simulink model "test2_Pace_UART"  (R2017b)
settings: Solver=FixedStepAuto  StartTime=0.0  StopTime=inf  FixedStep=1e-3  RelTol=1e-3  EnableMultiTasking=on
undefined symbols (not defined in the file): D0, D1, D10, D11, D12, D13, D2, D3, D5, D6, D8, D9, PTA0, PTA1, PTA2, PTB9, PTC16, PTC17, PTC2, PTC4, PTD0, PTD1, PTD2, PTD3
libraries: frdmk64flib x17, etargetslib x3
settings Model: ExtModeTrigDuration=5  Creator=zhuh30  LastModifiedBy=Michael
settings OptimizationCC: PassReuseOutputArgsAs=Individual arguments  MaxStackSize=64
settings DebuggingCC: ParameterTunabilityLossMsg=error
settings HardwareCC: ProdBitPerPointer=32  ProdBitPerSizeT=32  ProdBitPerPtrDiffT=32  ProdLargestAtomicInteger=Long  ProdLargestAtomicFloat=Double  ProdWordSize=32  ProdHWDeviceType=ARM Compatible->ARM Cortex
settings SFSimCC: MATLABDynamicMemAlloc=off
settings RTWCC: SystemTargetFile=ert.tlc  HardwareBoard=NXP FRDM-K64F  TemplateMakefile=ert_default_tmf  GenerateReport=on  Toolchain=GNU Tools for ARM Embedded Processors  IncludeHyperlinkInReport=on  LaunchReport=on  GenerateTraceInfo=on  GenerateTraceReport=on  GenerateTraceReportSl=on  GenerateTraceReportSf=on  GenerateTraceReportEml=on
settings CodeAppCC: ForceParamTrailComments=on  IgnoreCustomStorageClasses=off  OperatorAnnotations=on  SimulinkDataObjDesc=on  SFDataObjDesc=on  InsertBlockDesc=on

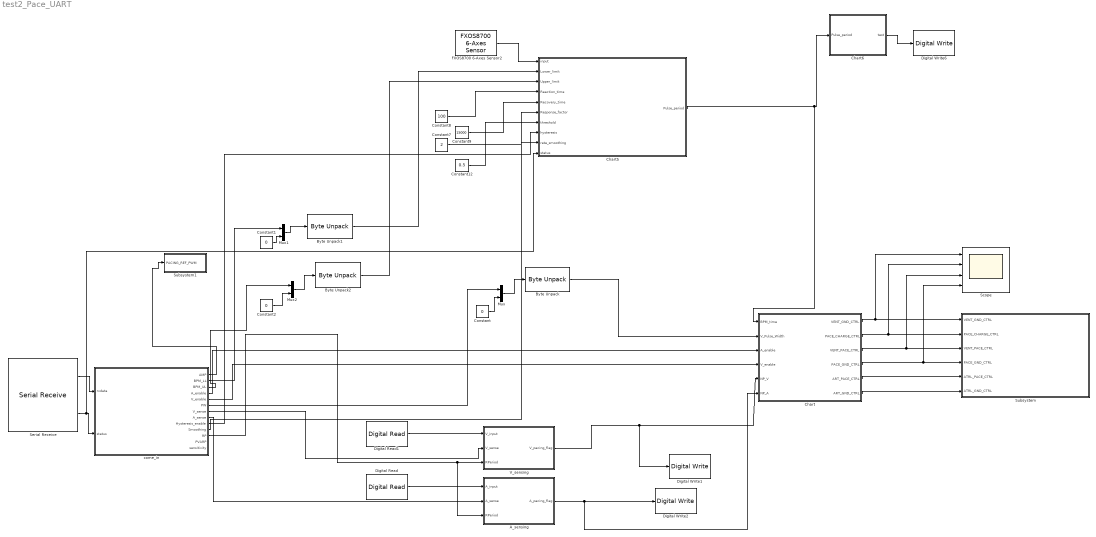
== system test2_Pace_UART ==
  A_sensing : Stateflow chart  TreatAsAtomicUnit=on
  Byte Unpack : etargetslib/Byte Unpack  dimensions={[1]}  datatypes={'uint16'}  byteAlign=1
  Byte Unpack1 : etargetslib/Byte Unpack  dimensions={[1]}  datatypes={'uint16'}  byteAlign=1
  Byte Unpack2 : etargetslib/Byte Unpack  dimensions={[1]}  datatypes={'uint16'}  byteAlign=1
  Chart : Stateflow chart  TreatAsAtomicUnit=on
  Chart5 : Stateflow chart  TreatAsAtomicUnit=on
  Chart6 : Stateflow chart  TreatAsAtomicUnit=on
  Constant : Constant  Value=0  OutDataTypeStr=uint8
  Constant1 : Constant  Value=0  OutDataTypeStr=uint8
  Constant12 : Constant  Value=0.5
  Constant2 : Constant  Value=0  OutDataTypeStr=uint8
  Constant7 : Constant  Value=2
  Constant8 : Constant  Value=100
  Constant9 : Constant  Value=15000
  Digital Read : frdmk64flib/Digital Read  Whichpin=PTC16 (D0)  SampleTime=-1
      settings: SourceProductName=Simulink Coder Support Package for NXP FRDM-K64F Board
  Digital Read1 : frdmk64flib/Digital Read  Whichpin=PTC17 (D1)  SampleTime=-1
      settings: SourceProductName=Simulink Coder Support Package for NXP FRDM-K64F Board
  Digital Write1 : frdmk64flib/Digital Write  Whichpin=RED_LED
      settings: SourceProductName=Simulink Coder Support Package for NXP FRDM-K64F Board
  Digital Write2 : frdmk64flib/Digital Write  Whichpin=BLUE_LED
      settings: SourceProductName=Simulink Coder Support Package for NXP FRDM-K64F Board
  Digital Write6 : frdmk64flib/Digital Write  Whichpin=GREEN_LED
      settings: SourceProductName=Simulink Coder Support Package for NXP FRDM-K64F Board
  FXOS8700 6-Axes Sensor2 : frdmk64flib/FXOS8700 6-Axes Sensor  Activesensor=Accelerometer only  ODR=800Hz  HybridODR=400Hz  Accelfullrange=-4g to +4g  SampleTime=-1
      settings: SourceProductName=Simulink Coder Support Package for NXP FRDM-K64F Board
  Mux : Mux  Inputs=2
  Mux1 : Mux  Inputs=2
  Mux2 : Mux  Inputs=2
  Scope : Scope  NumInputPorts=4
  Serial Receive : frdmk64flib/Serial Receive  SCIModule=0  Baudrate=uint32(9600)  Parity=None  StopBits=1  HardwareFlowControl=None  ByteOrder=LittleEndian  DataType=uint8  DataLength=15  BlockingMode=off  OutputStatus=on  SampleTime=-1
      settings: SourceProductName=Simulink Coder Support Package for NXP FRDM-K64F Board
  Subsystem : Subsystem
  Subsystem1 : Subsystem
  V_sensing : Stateflow chart  TreatAsAtomicUnit=on
  come_in : Stateflow chart  TreatAsAtomicUnit=on
  wires:
  come_in/1(AMP) -> Subsystem1/1(PACING_REF_PWM)
  Serial Receive/1 -> come_in/1(rxdata)
  Serial Receive/2 -> Chart5/10(status), come_in/2(status)
  come_in/2(BPM_LL) -> Mux1/1
  come_in/3(BPM_UL) -> Mux2/1
  come_in/6(PW) -> Mux/1
  Constant/1 -> Mux/2
  Mux/1 -> Byte Unpack/1
  Mux1/1 -> Byte Unpack1/1
  Constant1/1 -> Mux1/2
  Mux2/1 -> Byte Unpack2/1
  Constant2/1 -> Mux2/2
  V_sensing/1(V_pacing_flag) -> Digital Write1/1, Chart/5(NP_V)
  Digital Read/1 -> A_sensing/1(A_input)
  A_sensing/1(A_pacing_flag) -> Chart/6(NP_A), Digital Write2/1
  come_in/7(V_sense) -> V_sensing/2(V_sense)
  come_in/8(A_sense) -> A_sensing/2(A_sense)
  come_in/11(RP) -> A_sensing/3(RPeriod), V_sensing/3(RPeriod)
  Chart/5(ART_PACE_CTRL) -> Subsystem/5(ATRL_PACE_CTRL)
  Chart/3(VENT_PACE_CTRL) -> Scope/3, Subsystem/3(VENT_PACE_CTRL)
  Chart/6(ART_GND_CTRL) -> Subsystem/6(ATRL_GND_CTRL)
  Chart/1(VENT_GND_CTRL) -> Scope/1, Subsystem/1(VENT_GND_CTRL)
  Chart/2(PACE_CHARGE_CTRL) -> Scope/2, Subsystem/2(PACE_CHARGE_CTRL)
  Byte Unpack/1 -> Chart/2(V_Pulse_Width)
  Chart/4(PACE_GND_CTRL) -> Scope/4, Subsystem/4(PACE_GND_CTRL)
  Digital Read1/1 -> V_sensing/1(V_input)
  Byte Unpack2/1 -> Chart5/3(Upper_limit)
  FXOS8700 6-Axes Sensor2/1 -> Chart5/1(input)
  Constant12/1 -> Chart5/7(threshold)
  Byte Unpack1/1 -> Chart5/2(Lower_limit)
  Chart6/1(test) -> Digital Write6/1
  Constant9/1 -> Chart5/5(Recovery_time)
  Constant8/1 -> Chart5/4(Reaction_time)
  Constant7/1 -> Chart5/6(Response_factor)
  come_in/5(V_enable) -> Chart/4(V_enable)
  come_in/4(A_enable) -> Chart/3(A_enable)
  Chart5/1(Pulse_period) -> Chart/1(BPM_time), Chart6/1(Pulse_period)
  come_in/9(Hysteresis_enable) -> Chart5/8(hysteresis)
  come_in/10(Smoothing) -> Chart5/9(rate_smoothing)

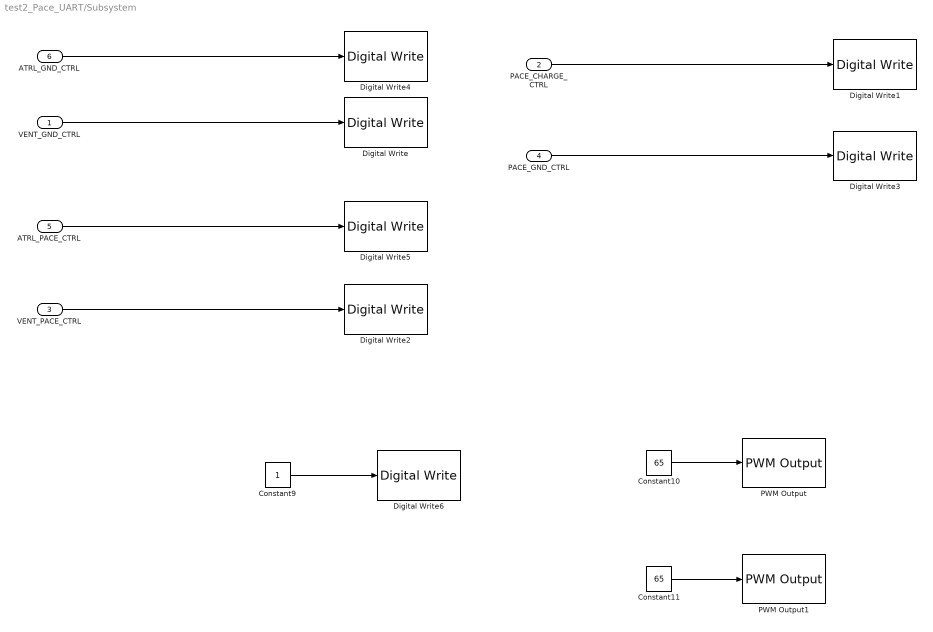
== system test2_Pace_UART/Subsystem ==
  VENT_GND_CTRL : Inport
  PACE_CHARGE_CTRL : Inport  Port=2
  VENT_PACE_CTRL : Inport  Port=3
  PACE_GND_CTRL : Inport  Port=4
  ATRL_PACE_CTRL : Inport  Port=5
  ATRL_GND_CTRL : Inport  Port=6
  Constant10 : Constant  Value=65
  Constant11 : Constant  Value=65
  Constant9 : Constant
  Digital Write : frdmk64flib/Digital Write  Whichpin=PTD3 (D12)
      settings: SourceProductName=Simulink Coder Support Package for NXP FRDM-K64F Board
  Digital Write1 : frdmk64flib/Digital Write  Whichpin=PTB9 (D2)
      settings: SourceProductName=Simulink Coder Support Package for NXP FRDM-K64F Board
  Digital Write2 : frdmk64flib/Digital Write  Whichpin=PTC4 (D9)
      settings: SourceProductName=Simulink Coder Support Package for NXP FRDM-K64F Board
  Digital Write3 : frdmk64flib/Digital Write  Whichpin=PTD0 (D10)
      settings: SourceProductName=Simulink Coder Support Package for NXP FRDM-K64F Board
  Digital Write4 : frdmk64flib/Digital Write  Whichpin=PTD2 (D11)
      settings: SourceProductName=Simulink Coder Support Package for NXP FRDM-K64F Board
  Digital Write5 : frdmk64flib/Digital Write  Whichpin=PTA0 (D8)
      settings: SourceProductName=Simulink Coder Support Package for NXP FRDM-K64F Board
  Digital Write6 : frdmk64flib/Digital Write  Whichpin=PTD1 (D13)
      settings: SourceProductName=Simulink Coder Support Package for NXP FRDM-K64F Board
  PWM Output : frdmk64flib/PWM Output  Whichpin=PTC2 (D6)  InitialFrequency=916  InitialDutyCycle=60
      settings: SourceProductName=Simulink Coder Support Package for NXP FRDM-K64F Board
  PWM Output1 : frdmk64flib/PWM Output  Whichpin=PTA1 (D3)  InitialFrequency=916  InitialDutyCycle=60
      settings: SourceProductName=Simulink Coder Support Package for NXP FRDM-K64F Board
  wires:
  VENT_GND_CTRL/1 -> Digital Write/1
  PACE_CHARGE_CTRL/1 -> Digital Write1/1
  VENT_PACE_CTRL/1 -> Digital Write2/1
  PACE_GND_CTRL/1 -> Digital Write3/1
  ATRL_GND_CTRL/1 -> Digital Write4/1
  ATRL_PACE_CTRL/1 -> Digital Write5/1
  Constant9/1 -> Digital Write6/1
  Constant10/1 -> PWM Output/1
  Constant11/1 -> PWM Output1/1

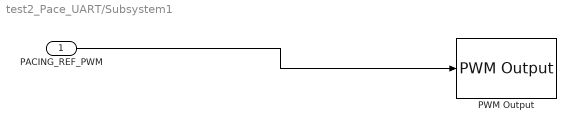
== system test2_Pace_UART/Subsystem1 ==
  PACING_REF_PWM : Inport
  PWM Output : frdmk64flib/PWM Output  Whichpin=PTA2 (D5)  InitialFrequency=916  InitialDutyCycle=0
      settings: SourceProductName=Simulink Coder Support Package for NXP FRDM-K64F Board
  wires:
  PACING_REF_PWM/1 -> PWM Output/1

== stateflow chart test2_Pace_UART/come_in ==
  state SET_RARAM [commented out]
    entry:
    BPM_UL = rxdata(3);
    BPM_LL = rxdata(4);
    AMP = rxdata(5);
    PW = rxdata(6);
  state INITIAL [commented out]
    entry:
    BPM_UL = 60;
    BPM_LL = 60;
    AMP = 60;
    PW = 100;
    A_enable = 1;
    V_enable = 0;
    A_sense = 1;
    V_sense = 0;
    RP = 500;
    Hysteresis_enable = 0;
    Smoothing = 0;
    PVARP = 0;
  state STANDBY [commented out]
  state SET_RARAM1
    entry:
    BPM_LL = rxdata(3);
    BPM_UL = rxdata(4);
    AMP = rxdata(5);
    PW = rxdata(6);
    if (rxdata(7) == hex2dec('1'))
    A_enable = 1;
    V_enable = 0;
    V_sense= 0;
    A_sense = rxdata(8);
    sensitivity = rxdata(9);
    RP = 10* typecast(rxdata(10:11), 'uint16');
    Hysteresis_enable = rxdata(12);
    Smoothing = rxdata(13);
    PVARP = typecast(rxdata(14:15), 'uint16');
    elseif (rxdata(7) == hex2dec('0'))
    A_enable = 0;
    V_enable = 1;
    A_sense= 0;
    V_sense = rxdata(8);
    sensitivity = rxdata(9);
    RP = 10*typecast(rxdata(10:11), 'uint16');
    Hysteresis_enable = rxdata(12);
    Smoothing = rxdata(13);
    PVARP = typecast(rxdata(14:15), 'uint16');
    else
    A_enable = 0;
    V_enable = 0;
    A_sense= 0;
    V_sense = rxdata(8);
    sensitivity = rxdata(9);
    RP = 10*typecast(rxdata(10:11), 'uint16');
    Hysteresis_enable = rxdata(12);
    Smoothing = rxdata(13);
    PVARP = typecast(rxdata(14:15), 'uint16');
    end
  state VOO_or_VVI [commented out]
    entry:
    A_enable = 0;
    V_enable = 1;
    A_sense = 0;
    V_sense = rxdata(8);
    sensitivity = rxdata(9);
    RP = 10*typecast(rxdata(10:11), 'uint16');
    Hysteresis_enable = rxdata(12);
    Smoothing = rxdata(13);
    PVARP = typecast(rxdata(14:15), 'uint16');
  state AOO_or_AAI [commented out]
    entry:
    A_enable = 1;
    V_enable = 0;
    V_sense = 0;
    A_sense = rxdata(8);
    sensitivity = rxdata(9);
    RP = 10* typecast(rxdata(10:11), 'uint16');
    Hysteresis_enable = rxdata(12);
    Smoothing = rxdata(13);
    PVARP = typecast(rxdata(14:15), 'uint16');
  state INITIAL1
    entry:
    BPM_UL = 120;
    BPM_LL = 60;
    AMP = 60;
    PW = 100;
    A_enable = 1;
    V_enable = 0;
    A_sense = 1;
    V_sense = 0;
    RP = 50;
    Hysteresis_enable = 0;
    Smoothing = 0;
    PVARP = 0;
  state STANDBY1
  SET_RARAM -> STANDBY [commented out]
  (junction 6) -> STANDBY [commented out]
  (default) -> INITIAL [commented out]
  INITIAL -> STANDBY [commented out]
  STANDBY -> (junction 6) [commented out] : [status == 0]
  (junction 6) -> (junction 7) [commented out] : [rxdata(1) == hex2dec('16')]
  (junction 7) -> SET_RARAM [commented out] : [rxdata(2) == hex2dec('55')]
  (junction 7) -> STANDBY [commented out]
  VOO_or_VVI -> STANDBY [commented out]
  AOO_or_AAI -> STANDBY [commented out]
  SET_RARAM -> AOO_or_AAI [commented out] : [rxdata(7) == hex2dec('1')]
  SET_RARAM -> VOO_or_VVI [commented out] : [rxdata(7) == hex2dec('0')]
  (junction 55) -> STANDBY1 [order 2]
  (default) -> INITIAL1
  INITIAL1 -> STANDBY1
  STANDBY1 -> (junction 55) : [status == 0]
  (junction 55) -> (junction 63) [order 1] : [rxdata(1) == hex2dec('16')]
  (junction 63) -> SET_RARAM1 [order 1] : [rxdata(2) == hex2dec('55')]
  (junction 63) -> STANDBY1 [order 2]
  SET_RARAM1 -> STANDBY1
  data: AMP output uint8; rxdata input uint8; status input uint8; BPM_LL output uint8; BPM_UL output uint8; A_enable output uint8; V_enable output uint8; PW output uint8; V_sense output uint8; A_sense output uint8; Hysteresis_enable output uint8; Smoothing output uint8; RP output uint16; PVARP output uint16; sensitivity output uint8

== stateflow chart test2_Pace_UART/A_sensing ==
  state SENSING_A_wait
    entry:
    A_pacing_flag = 0;
  state A_pace_sensed
    entry:
    A_pacing_flag = 1;
  SENSING_A_wait -> A_pace_sensed [order 2] : [A_input == 1]
  (default) -> SENSING_A_wait
  A_pace_sensed -> SENSING_A_wait : after(RPeriod,msec)
  SENSING_A_wait -> SENSING_A_wait [order 1] : [A_sense == 0]
  data: A_input input; A_pacing_flag output uint8; A_sense input; RPeriod input

== stateflow chart test2_Pace_UART/Chart ==
  state Initial_state
    entry:
    ART_PACE_CTRL = false;
    ART_GND_CTRL = true
    VENT_PACE_CTRL = false;
    VENT_GND_CTRL = true;
    PACE_CHARGE_CTRL = true;
    PACE_GND_CTRL = true;
  state Charging_state_V
    entry:
    PACE_CHARGE_CTRL = true;
    VENT_PACE_CTRL = false;
    VENT_GND_CTRL = true;
    PACE_GND_CTRL = true;
    ART_PACE_CTRL = false;
    ART_GND_CTRL = true;
  state Charging_state_A
    entry:
    PACE_CHARGE_CTRL = true;
    ART_PACE_CTRL = false;
    ART_GND_CTRL = true;
    PACE_GND_CTRL = true;
    VENT_PACE_CTRL = false;
    VENT_GND_CTRL = true;
  state Delay_state_A
    entry:
    PACE_CHARGE_CTRL = true;
    ART_PACE_CTRL = false;
    ART_GND_CTRL = true;
    PACE_GND_CTRL = true;
    VENT_PACE_CTRL = false;
    VENT_GND_CTRL = true;
  state Delay_state_V
    entry:
    PACE_CHARGE_CTRL = true;
    VENT_PACE_CTRL = false;
    VENT_GND_CTRL = true;
    PACE_GND_CTRL = true;
    ART_PACE_CTRL = false;
    ART_GND_CTRL = true;
  state Pacing_state_V
    entry:
    PACE_CHARGE_CTRL = false;
    VENT_PACE_CTRL = true;
    VENT_GND_CTRL = false;
    PACE_GND_CTRL = true;
    ART_PACE_CTRL = false;
    ART_GND_CTRL = true;
  state Pacing_state
    entry:
    PACE_CHARGE_CTRL = false;
    ART_PACE_CTRL = true;
    ART_GND_CTRL = false;
    PACE_GND_CTRL = true;
    VENT_PACE_CTRL = false;
    VENT_GND_CTRL = true;
  (default) -> Initial_state
  Initial_state -> Charging_state_V [order 1] : [V_enable == 1]
  Initial_state -> Charging_state_A [order 2] : [A_enable == 1]
  Charging_state_A -> Delay_state_A [order 2] : [NP_A == 1]
  Charging_state_V -> Delay_state_V [order 2] : [NP_V == 1]
  Charging_state_V -> Charging_state_A [order 3] : [A_enable == 1]
  Delay_state_A -> Delay_state_A [order 1] : [NP_A == 1]
  Charging_state_A -> Charging_state_V [order 3] : [V_enable == 1]
  Delay_state_V -> Delay_state_V [order 1] : [NP_V == 1]
  Pacing_state -> Charging_state_A [order 1] : after(V_Pulse_Width,msec)
  Pacing_state_V -> Charging_state_V [order 1] : after(V_Pulse_Width,msec)
  Charging_state_V -> Pacing_state_V [order 1] : after(BPM_time-V_Pulse_Width,msec)
  Charging_state_A -> Pacing_state [order 1] : after(BPM_time-V_Pulse_Width,msec)
  Delay_state_A -> Pacing_state [order 2] : after(BPM_time,msec)
  Pacing_state -> Delay_state_A [order 2] : [NP_A == 1]
  Delay_state_V -> Pacing_state_V [order 2] : after(BPM_time,msec)
  Pacing_state_V -> Delay_state_V [order 2] : [NP_V == 1]
  data: BPM_time input; VENT_GND_CTRL output; PACE_CHARGE_CTRL output; VENT_PACE_CTRL output; PACE_GND_CTRL output; V_Pulse_Width input; A_enable input; V_enable input; ART_PACE_CTRL output; ART_GND_CTRL output; NP_V input; NP_A input

== stateflow chart test2_Pace_UART/V_sensing ==
  state SENSING_V_wait
    entry:
    V_pacing_flag = 0;
  state V_pacing_sensed
    entry:
    V_pacing_flag = 1;
  SENSING_V_wait -> V_pacing_sensed [order 2] : [V_input == 1]
  (default) -> SENSING_V_wait
  V_pacing_sensed -> SENSING_V_wait : after(RPeriod,msec)
  SENSING_V_wait -> SENSING_V_wait [order 1] : [V_sense == 0]
  data: V_input input; V_pacing_flag output uint8; V_sense input; RPeriod input

== stateflow chart test2_Pace_UART/Chart5 ==
  state Initial1
    entry:
    norm_xy = ((input(1)^2.0) + (input(2)^2.0))^(1/2);
    BPM = Lower_limit;
    Pulse_period = uint16(60000/BPM);
    counter_reaction = 0;
    counter_recovery = 0;
  state norm_over_state
    entry:
    norm_xy = ((input(1)^2.0) + (input(2)^2.0))^(1/2);
    counter_reaction = counter_reaction + 1;
    counter_recovery = 0;
    counter_update_increase = 0;
  state norm_below_state
    entry:
    if (BPM > (Lower_limit + Upper_limit)/2)
    BPM = BPM - Response_factor;
    else
    BPM = Lower_limit;
    end
    Pulse_period = uint16(60000/BPM);
    norm_xy = ((input(1)^2.0) + (input(2)^2.0))^(1/2);
    counter_update = 0;
    counter_reaction = 0;
    counter_recovery = counter_recovery + 1;
  state update_input
    entry:
    norm_xy = ((input(1)^2.0) + (input(2)^2.0))^(1/2);
    counter_update = counter_update + 1;
    counter_update_increase = 0;
  state update_input_increase
    entry:
    norm_xy = ((input(1)^2.0) + (input(2)^2.0))^(1/2);
    counter_update_increase=counter_update_increase + 1;
  state Increase_rate
    entry:
    if (BPM < Upper_limit)
    BPM = BPM + Response_factor;
    else
    BPM = Upper_limit;
    end
    Pulse_period = uint16(60000/BPM);
    norm_xy = ((input(1)^2.0) + (input(2)^2.0))^(1/2);
    counter_reaction = 0;
    counter_update_increase = 0;
    counter_update = 0;
    counter_recovery = 0;
  Initial1 -> Initial1 [order 2] : after(1,msec)
  (default) -> Initial1
  Initial1 -> norm_over_state [order 1] : [norm_xy>threshold]
  norm_below_state -> Initial1 [order 2] : [counter_recovery >= 30]
  norm_over_state -> Initial1 [order 2] : [norm_xy <= threshold]
  norm_below_state -> Initial1 [order 1] : [status == 0]
  norm_over_state -> Initial1 [order 1] : [status == 0]
  update_input_increase -> Initial1 [order 1] : [status == 0]
  Increase_rate -> Initial1 [order 1] : [status == 0]
  update_input -> Initial1 [order 1] : [status == 0]
  norm_over_state -> norm_over_state [order 4] : after(1,msec)
  norm_below_state -> norm_over_state [order 3] : [norm_xy > threshold]
  update_input -> norm_over_state [order 4] : [norm_xy > threshold]
  norm_over_state -> update_input_increase [order 3] : [counter_reaction >= Reaction_time]
  norm_below_state -> update_input [order 4] : [norm_xy <= threshold]
  update_input -> norm_below_state [order 2] : [counter_update >= Recovery_time/30]
  update_input_increase -> update_input [order 3] : [norm_xy <= threshold]
  update_input -> update_input [order 3] : after(1,msec)
  Increase_rate -> update_input [order 2] : [norm_xy <= threshold]
  Increase_rate -> update_input_increase [order 3] : [norm_xy > threshold]
  update_input_increase -> Increase_rate [order 2] : [counter_update_increase >= 250]
  update_input_increase -> update_input_increase [order 4] : after(1,msec)
  data: input input; Lower_limit input; Upper_limit input; Pulse_period output; Reaction_time input; Recovery_time input; Response_factor input; norm_xy local; BPM local; threshold input; hysteresis input; rate_smoothing input; counter_reaction local; counter_update local; counter_recovery local; counter_update_increase local; status input

== stateflow chart test2_Pace_UART/Chart6 ==
  state state
    entry:
    if (Pulse_period > 856)
    test = false;
    else
    test = true;
    end
  (default) -> state
  state -> state : after(1,msec)
  data: test output boolean; Pulse_period input uint16
